simulink model "PID"  (R2019a)
settings: Solver=VariableStepAuto  StartTime=0.0  StopTime=10.0  RelTol=1e-3
values from neighbouring files (symbols this model uses):
  kd = kp*Td    (= 7.5)    [Compensator.m]
  ki = kp/Ti    (= 1.2)    [Compensator.m]
  kp = 0.6*Kpid    (= 6)    [Compensator.m]
undefined symbols (not defined in the file or in its folder): den, num
settings Model: Creator=xde12  LastModifiedBy=xde12

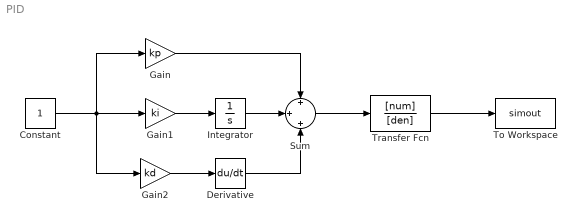
== system PID ==
  Constant : Constant
  Derivative : Derivative
  Gain : Gain  Gain=kp
  Gain1 : Gain  Gain=ki
  Gain2 : Gain  Gain=kd
  Integrator : Integrator
  Sum : Sum  Inputs=+|+|+
  To Workspace : ToWorkspace  VariableName=simout  SaveFormat=Timeseries  SampleTime=-1
  Transfer Fcn : TransferFcn  Numerator=[num]  Denominator=[den]
  wires:
  Constant/1 -> Gain2/1, Gain/1, Gain1/1
  Gain1/1 -> Integrator/1
  Integrator/1 -> Sum/2
  Gain/1 -> Sum/1
  Gain2/1 -> Derivative/1
  Derivative/1 -> Sum/3
  Sum/1 -> Transfer Fcn/1
  Transfer Fcn/1 -> To Workspace/1
